simulink model "stcd_CSII"  (Simulink 7.5)
settings: Solver=ode45  StartTime=0.0  StopTime=10.0  RelTol=1e-3
undefined symbols (not defined in the file or in its folder): ctrller
settings Model: Creator=sriddle  LastModifiedBy=sriddle

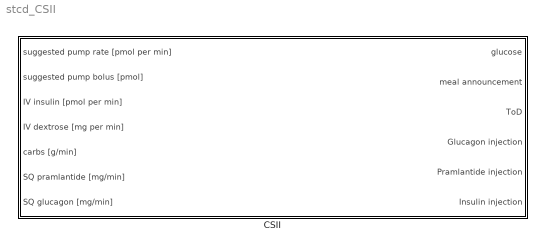
== system stcd_CSII ==
  CSII : Subsystem

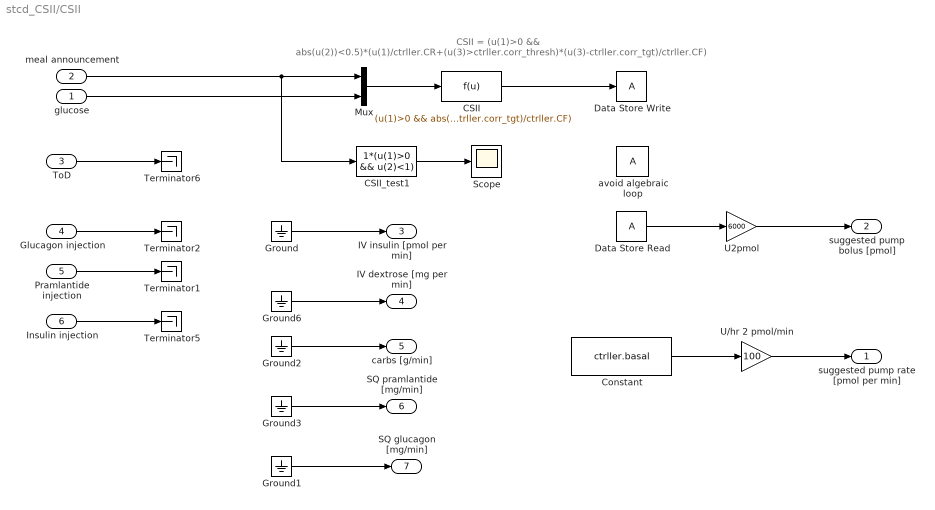
== system stcd_CSII/CSII ==
  note: CSII = (u(1)>0 && abs(u(2))<0.5)*(u(1)/ctrller.CR+(u(3)>ctrller.corr_thresh)*(u(3)-ctrller.corr_tgt)/ctrller.CF)
  glucose : Inport
  meal announcement : Inport  Port=2
  ToD : Inport  Port=3
  Glucagon injection : Inport  Port=4
  Pramlantide injection : Inport  Port=5
  Insulin injection : Inport  Port=6
  CSII : Fcn  Expr=(u(1)>0 && abs(u(2))<0.5)*(u(1)/ctrller.CR+(u(3)>ctrller.corr_thresh)*(u(3)-ctrller.corr_tgt)/ctrller.CF)  SampleTime=1
  CSII_test1 : Fcn  Expr=1*(u(1)>0 && u(2)<1)  SampleTime=1
  Constant : Constant  Value=ctrller.basal  OutDataType=fixdt(1, 16)  OutScaling=2^0
  Data Store Read : DataStoreRead  DataStoreName=A  SampleTime=1
  Data Store Write : DataStoreWrite  DataStoreName=A  SampleTime=1
  Ground{,1..3,6} (5 alike) : Ground
  Mux : Mux  Inputs=2
  Scope : Scope
      settings: SaveName=ScopeData9
  Terminator{1..2,5..6} (4 alike) : Terminator
  U/hr 2 pmol/min : Gain  Gain=100  ParameterDataType=fixdt(1, 16)  ParameterScaling=2^0  OutDataType=fixdt(1, 16)  OutScaling=2^0  SampleTime=1
  U2pmol : Gain  Gain=6000  ParameterDataType=fixdt(1, 16)  ParameterScaling=2^0  OutDataType=fixdt(1, 16)  OutScaling=2^0  SampleTime=1
  avoid algebraic loop : DataStoreMemory  DataStoreName=A  ReadBeforeWriteMsg=warning  WriteAfterWriteMsg=warning  WriteAfterReadMsg=warning  OutDataType=fixdt(1, 16)  OutScaling=2^0
  suggested pump rate [pmol per min] : Outport
  suggested pump bolus [pmol] : Outport  Port=2
  IV insulin [pmol per min] : Outport  Port=3
  IV dextrose [mg per min] : Outport  Port=4
  carbs [g/min] : Outport  Port=5
  SQ pramlantide [mg/min] : Outport  Port=6
  SQ glucagon [mg/min] : Outport  Port=7
  wires:
  Glucagon injection/1 -> Terminator2/1
  Pramlantide injection/1 -> Terminator1/1
  Ground/1 -> IV insulin [pmol per min]/1
  Ground1/1 -> SQ glucagon [mg/min]/1
  Ground3/1 -> SQ pramlantide [mg/min]/1
  Ground2/1 -> carbs [g/min]/1
  glucose/1 -> Mux/2
  Insulin injection/1 -> Terminator5/1
  ToD/1 -> Terminator6/1
  Constant/1 -> U/hr 2 pmol/min/1
  Ground6/1 -> IV dextrose [mg per min]/1
  Data Store Read/1 -> U2pmol/1
  U2pmol/1 -> suggested pump bolus [pmol]/1
  CSII/1 -> Data Store Write/1
  U/hr 2 pmol/min/1 -> suggested pump rate [pmol per min]/1
  meal announcement/1 -> Mux/1, CSII_test1/1
  CSII_test1/1 -> Scope/1
  Mux/1 -> CSII/1
